simulink model "Limitatore"  (R2024b)
settings: Solver=VariableStepAuto  StartTime=0.0  StopTime=10  RelTol=1e-3
undefined symbols (not defined in the file or in its folder): ia_limite, kamp, klim, kt, kv, Vctr, Vnom
libraries: cstblocks x2
settings Model: Creator=turco  LastModifiedBy=turco

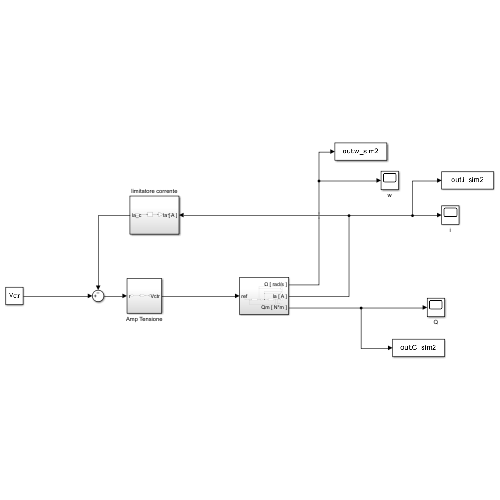
[thumbnail: Simulink's stored preview of the top-level diagram]
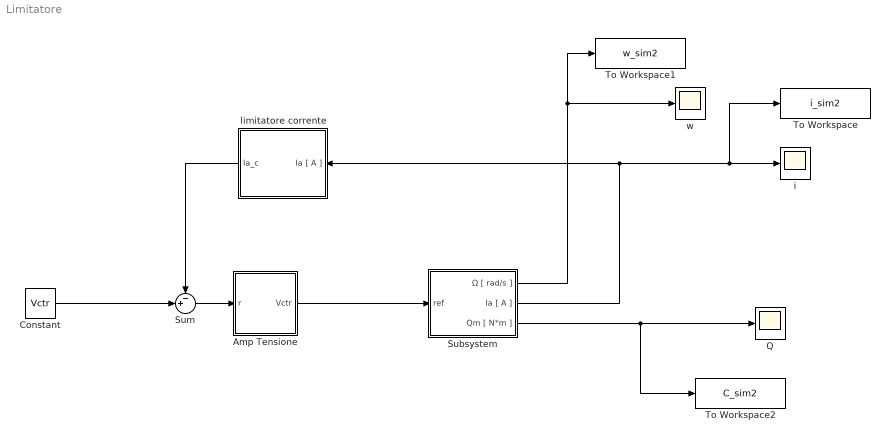
== system Limitatore ==
  Amp Tensione : Subsystem
  Constant : Constant  Value=Vctr
  Q : Scope
  Subsystem : Subsystem
  Sum : Sum  Inputs=-+|
  To Workspace : ToWorkspace  VariableName=i_sim2  SaveFormat=Timeseries  SampleTime=-1
  To Workspace1 : ToWorkspace  VariableName=w_sim2  SaveFormat=Timeseries  SampleTime=-1
  To Workspace2 : ToWorkspace  VariableName=C_sim2  SaveFormat=Timeseries  SampleTime=-1
  i : Scope
  limitatore corrente : Subsystem
  w : Scope
  wires:
  limitatore corrente/1(Ia_c) -> Sum/1
  Subsystem/2(Ia [ A ]) -> To Workspace/1, i/1, limitatore corrente/1(Ia [ A ])
  Amp Tensione/1(Vctr) -> Subsystem/1(ref)
  Sum/1 -> Amp Tensione/1(r)
  Subsystem/3(Qm [ N*m ]) -> To Workspace2/1, Q/1
  Subsystem/1(Ω [ rad/s ]) -> To Workspace1/1, w/1
  Constant/1 -> Sum/2

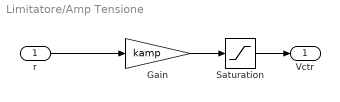
== system Limitatore/Amp Tensione ==
  r : Inport
  Gain : Gain  Gain=kamp
  Saturation : Saturate  UpperLimit=+Vnom*1.2  LowerLimit=-Vnom*1.2
  Vctr : Outport
  wires:
  r/1 -> Gain/1
  Saturation/1 -> Vctr/1
  Gain/1 -> Saturation/1

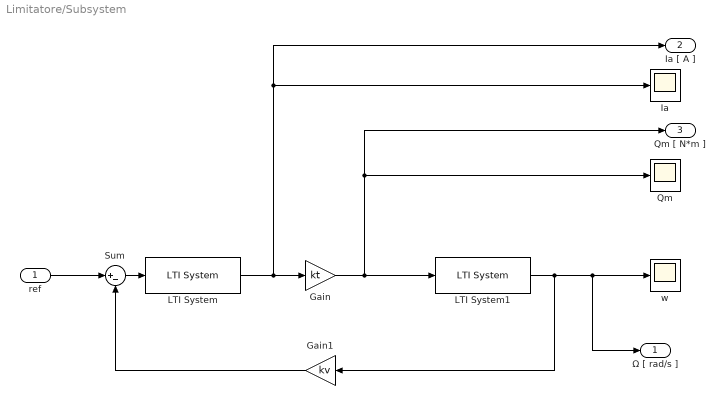
== system Limitatore/Subsystem ==
  ref : Inport
  Gain : Gain  Gain=kt
  Gain1 : Gain  Gain=kv
  Ia : Scope
  LTI System : cstblocks/LTI System  sys=Pel  IC=[]  PadeOrder=0
  LTI System1 : cstblocks/LTI System  sys=Pmec  IC=[]  PadeOrder=0
  "Qm " : Scope
  Sum : Sum  Inputs=|+-
  w : Scope
  Ω [ rad/s ] : Outport
  Ia [ A ] : Outport  Port=2
  Qm [ N*m ] : Outport  Port=3
  wires:
  LTI System1/1 -> Ω [ rad/s ]/1, w/1, Gain1/1
  Gain1/1 -> Sum/2
  Gain/1 -> Qm [ N*m ]/1, "Qm "/1, LTI System1/1
  Sum/1 -> LTI System/1
  LTI System/1 -> Ia [ A ]/1, Ia/1, Gain/1
  ref/1 -> Sum/1

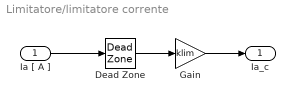
== system Limitatore/limitatore corrente ==
  Ia [ A ] : Inport
  Dead Zone : DeadZone  LowerValue=-ia_limite  UpperValue=+ia_limite
  Gain : Gain  Gain=klim
  Ia_c : Outport
  wires:
  Gain/1 -> Ia_c/1
  Ia [ A ]/1 -> Dead Zone/1
  Dead Zone/1 -> Gain/1
